simulink model "model"  (Simulink 9.1)
settings: Solver=VariableStepAuto  StartTime=0.0  StopTime=10.0  RelTol=1e-3
settings Model: Creator=User  LastModifiedBy=User
settings DataIOCC: SaveFormat=Dataset
settings OptimizationCC: LifeSpan=auto
settings DebuggingCC: UnderspecifiedInitializationDetection=Simplified  MergeDetectMultiDrivingBlocksExec=error  SFUnexpectedBacktrackingDiag=error  SFNoUnconditionalDefaultTransitionDiag=error  SFExecutionAtInitializationDiag=warning
settings HardwareCC: ProdBitPerPointer=64  ProdBitPerSizeT=64  ProdBitPerPtrDiffT=64  ProdLargestAtomicFloat=Float  ProdIntDivRoundTo=Zero  ProdEndianess=LittleEndian  ProdWordSize=64  ProdHWDeviceType=Intel->x86-64 (Windows64)
settings ModelReferenceCC: PropagateSignalLabelsOutOfModel=on
settings GRTTargetCC: TargetLangStandard=C99 (ISO)  CombineOutputUpdateFcns=on  GRTInterface=off
settings ConfigComp: CovMetricSettings=dwe  CovHtmlReporting=off  CovSaveCumulativeToWorkspaceVar=off  CovSaveSingleToWorkspaceVar=off  CovExternalEMLEnable=on

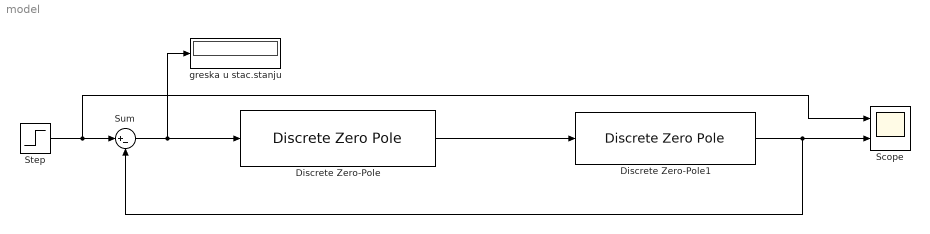
== system model ==
  Discrete Zero-Pole : DiscreteZeroPole  Zeros=[-0.8167]  Poles=[0.8187 0.6703]  Gain=0.0329  SampleTime=-1
  Discrete Zero-Pole1 : DiscreteZeroPole  Zeros=[0.6703 0.9145]  Poles=[0.3814 0.99]  Gain=5.485  SampleTime=-1
  Scope : Scope  NumInputPorts=2
  Step : Step  SampleTime=0
  Sum : Sum  Inputs=|+-
  "greska u stac.stanju " : Display
  wires:
  Discrete Zero-Pole/1 -> Discrete Zero-Pole1/1
  Step/1 -> Scope/1, Sum/1
  Sum/1 -> Discrete Zero-Pole/1, "greska u stac.stanju "/1
  Discrete Zero-Pole1/1 -> Sum/2, Scope/2
